simulink model "PulsePairProc"  (Simulink 6.4)
settings: Solver=ode45  StartTime=0.0  StopTime=40000/12e6  RelTol=1e-3
libraries: xbsIndex_r4 x256, simulink x2, dspsrcs4 x1
(part 2 of 2)

== system PulsePairProc/Pulse Pair Processor/Sum/A Avg/Avg. A 2 ==
  In : Inport
  M : Inport  Port=2
  N : Inport  Port=3
  Gate : Inport  Port=4
  Reset : Inport  Port=5
  AddSub2 : xbsIndex_r4/AddSub  mode=Addition  use_carryin=off  use_carryout=off  en=off  latency=0  precision=User Defined  arith_type="Signed  (2's comp)"  n_bits=33  bin_pt=31  quantization="Round  (unbiased: +/- Inf)"  overflow=Flag as error  dbl_ovrd=off  use_behavioral_HDL=off  pipelined=on  use_rpm=on  block_type=addsub
      settings: block_version=8.2
  Delay : xbsIndex_r4/Delay  en=off  latency=1  dbl_ovrd=off  reg_retiming=off  block_type=delay
      settings: infoedit=Hardware notes: A delay line is a chain, each link of which is an SRL16 followed by a flip-flop. If register retiming is enabled, the delay line is a chain of flip-flops.  block_version=8.2
  Delay1 : xbsIndex_r4/Delay  en=off  latency=1  dbl_ovrd=off  reg_retiming=off  block_type=delay
      settings: infoedit=Hardware notes: A delay line is a chain, each link of which is an SRL16 followed by a flip-flop. If register retiming is enabled, the delay line is a chain of flip-flops.  block_version=8.2
  FIFO : xbsIndex_r4/FIFO  depth=1K  percent_nbits=1  rst=on  en=off  dbl_ovrd=off  mem_type=Block RAM  block_type=fifo
      settings: block_version=8.2
  Logical : xbsIndex_r4/Logical  logical_function=OR  inputs=2  en=off  latency=0  precision=Full  arith_type=Unsigned  n_bits=16  bin_pt=0  align_bp=on  dbl_ovrd=off  block_type=logical
      settings: block_version=8.2
  Logical4 : xbsIndex_r4/Logical  logical_function=OR  inputs=2  en=off  latency=0  precision=Full  arith_type=Unsigned  n_bits=16  bin_pt=0  align_bp=on  dbl_ovrd=off  block_type=logical
      settings: block_version=8.2
  Mux : xbsIndex_r4/Mux  inputs=2  en=off  latency=0  precision=Full  arith_type=Unsigned  n_bits=16  bin_pt=14  quantization=Truncate  overflow=Wrap  dbl_ovrd=off  block_type=mux
      settings: block_version=8.2
  Register : xbsIndex_r4/Register  init=0  rst=on  en=on  dbl_ovrd=off  block_type=register
      settings: block_version=8.2
  Register1 : xbsIndex_r4/Register  init=0  rst=on  en=off  dbl_ovrd=off  block_type=register
      settings: block_version=8.2
  Shift : xbsIndex_r4/Shift  shift_dir=Right  shift_bits=1  en=off  latency=0  precision=User Defined  arith_type="Signed  (2's comp)"  n_bits=32  bin_pt=31  quantization="Round  (unbiased: +/- Inf)"  overflow=Flag as error  dbl_ovrd=off  block_type=shift
      settings: block_version=8.2
  Subsystem : Subsystem
  Out : Outport
  A,B,P Gate 1 : Outport  Port=2
  wires:
  Subsystem/1(WE) -> FIFO/2
  Subsystem/2(RE) -> Register1/1, FIFO/3
  Mux/1 -> FIFO/1, Register/1
  AddSub2/1 -> Shift/1
  FIFO/1 -> AddSub2/1
  Register1/1 -> Mux/1
  In/1 -> Delay/1
  Register/1 -> Out/1
  M/1 -> Subsystem/2(M)
  Subsystem/4(Out_En) -> Register/3, Delay1/1, Logical/2
  N/1 -> Subsystem/3(N)
  Delay/1 -> Mux/2, AddSub2/2
  Gate/1 -> Subsystem/1(Enable)
  Delay1/1 -> Logical/1
  Logical/1 -> A,B,P Gate 1/1
  Reset/1 -> Subsystem/4(Reset), Logical4/2, FIFO/4
  Logical4/1 -> Register1/2, Register/2
  Subsystem/3(RST) -> Logical4/1
  Shift/1 -> Mux/3

== system PulsePairProc/Pulse Pair Processor/Sum/B Avg/Avg. B 1 ==
  In : Inport
  M : Inport  Port=2
  N : Inport  Port=3
  Gate : Inport  Port=4
  Reset : Inport  Port=5
  AddSub2 : xbsIndex_r4/AddSub  mode=Addition  use_carryin=off  use_carryout=off  en=off  latency=0  precision=User Defined  arith_type="Signed  (2's comp)"  n_bits=33  bin_pt=31  quantization="Round  (unbiased: +/- Inf)"  overflow=Flag as error  dbl_ovrd=off  use_behavioral_HDL=off  pipelined=on  use_rpm=on  block_type=addsub
      settings: block_version=8.2
  Delay : xbsIndex_r4/Delay  en=off  latency=1  dbl_ovrd=off  reg_retiming=off  block_type=delay
      settings: infoedit=Hardware notes: A delay line is a chain, each link of which is an SRL16 followed by a flip-flop. If register retiming is enabled, the delay line is a chain of flip-flops.  block_version=8.2
  FIFO : xbsIndex_r4/FIFO  depth=1K  percent_nbits=1  rst=on  en=off  dbl_ovrd=off  mem_type=Block RAM  block_type=fifo
      settings: block_version=8.2
  Logical4 : xbsIndex_r4/Logical  logical_function=OR  inputs=2  en=off  latency=0  precision=Full  arith_type=Unsigned  n_bits=16  bin_pt=0  align_bp=on  dbl_ovrd=off  block_type=logical
      settings: block_version=8.2
  Mux : xbsIndex_r4/Mux  inputs=2  en=off  latency=0  precision=Full  arith_type=Unsigned  n_bits=16  bin_pt=14  quantization=Truncate  overflow=Wrap  dbl_ovrd=off  block_type=mux
      settings: block_version=8.2
  Register : xbsIndex_r4/Register  init=0  rst=on  en=on  dbl_ovrd=off  block_type=register
      settings: block_version=8.2
  Register1 : xbsIndex_r4/Register  init=0  rst=on  en=off  dbl_ovrd=off  block_type=register
      settings: block_version=8.2
  Shift : xbsIndex_r4/Shift  shift_dir=Right  shift_bits=1  en=off  latency=0  precision=User Defined  arith_type="Signed  (2's comp)"  n_bits=32  bin_pt=31  quantization="Round  (unbiased: +/- Inf)"  overflow=Flag as error  dbl_ovrd=off  block_type=shift
      settings: block_version=8.2
  Subsystem : Subsystem
  Out : Outport
  wires:
  Subsystem/1(WE) -> FIFO/2
  Subsystem/2(RE) -> Register1/1, FIFO/3
  Mux/1 -> FIFO/1, Register/1
  AddSub2/1 -> Shift/1
  FIFO/1 -> AddSub2/1
  Register1/1 -> Mux/1
  In/1 -> Delay/1
  Register/1 -> Out/1
  M/1 -> Subsystem/2(M)
  Subsystem/4(Out_En) -> Register/3
  N/1 -> Subsystem/3(N)
  Delay/1 -> Mux/2, AddSub2/2
  Gate/1 -> Subsystem/1(Enable)
  Reset/1 -> Subsystem/4(Reset), Logical4/2, FIFO/4
  Logical4/1 -> Register1/2, Register/2
  Subsystem/3(RST) -> Logical4/1
  Shift/1 -> Mux/3

== system PulsePairProc/Pulse Pair Processor/Sum/B Avg/Avg. B 2 ==
  In : Inport
  M : Inport  Port=2
  N : Inport  Port=3
  Gate : Inport  Port=4
  Reset : Inport  Port=5
  AddSub2 : xbsIndex_r4/AddSub  mode=Addition  use_carryin=off  use_carryout=off  en=off  latency=0  precision=User Defined  arith_type="Signed  (2's comp)"  n_bits=33  bin_pt=31  quantization="Round  (unbiased: +/- Inf)"  overflow=Flag as error  dbl_ovrd=off  use_behavioral_HDL=off  pipelined=on  use_rpm=on  block_type=addsub
      settings: block_version=8.2
  Delay : xbsIndex_r4/Delay  en=off  latency=1  dbl_ovrd=off  reg_retiming=off  block_type=delay
      settings: infoedit=Hardware notes: A delay line is a chain, each link of which is an SRL16 followed by a flip-flop. If register retiming is enabled, the delay line is a chain of flip-flops.  block_version=8.2
  FIFO : xbsIndex_r4/FIFO  depth=1K  percent_nbits=1  rst=on  en=off  dbl_ovrd=off  mem_type=Block RAM  block_type=fifo
      settings: block_version=8.2
  Logical4 : xbsIndex_r4/Logical  logical_function=OR  inputs=2  en=off  latency=0  precision=Full  arith_type=Unsigned  n_bits=16  bin_pt=0  align_bp=on  dbl_ovrd=off  block_type=logical
      settings: block_version=8.2
  Mux : xbsIndex_r4/Mux  inputs=2  en=off  latency=0  precision=Full  arith_type=Unsigned  n_bits=16  bin_pt=14  quantization=Truncate  overflow=Wrap  dbl_ovrd=off  block_type=mux
      settings: block_version=8.2
  Register : xbsIndex_r4/Register  init=0  rst=on  en=on  dbl_ovrd=off  block_type=register
      settings: block_version=8.2
  Register1 : xbsIndex_r4/Register  init=0  rst=on  en=off  dbl_ovrd=off  block_type=register
      settings: block_version=8.2
  Shift : xbsIndex_r4/Shift  shift_dir=Right  shift_bits=1  en=off  latency=0  precision=User Defined  arith_type="Signed  (2's comp)"  n_bits=32  bin_pt=31  quantization="Round  (unbiased: +/- Inf)"  overflow=Flag as error  dbl_ovrd=off  block_type=shift
      settings: block_version=8.2
  Subsystem : Subsystem
  Out : Outport
  wires:
  Subsystem/1(WE) -> FIFO/2
  Subsystem/2(RE) -> Register1/1, FIFO/3
  Mux/1 -> FIFO/1, Register/1
  AddSub2/1 -> Shift/1
  FIFO/1 -> AddSub2/1
  Register1/1 -> Mux/1
  In/1 -> Delay/1
  Register/1 -> Out/1
  M/1 -> Subsystem/2(M)
  Subsystem/4(Out_En) -> Register/3
  N/1 -> Subsystem/3(N)
  Delay/1 -> Mux/2, AddSub2/2
  Gate/1 -> Subsystem/1(Enable)
  Reset/1 -> Subsystem/4(Reset), Logical4/2, FIFO/4
  Logical4/1 -> Register1/2, Register/2
  Subsystem/3(RST) -> Logical4/1
  Shift/1 -> Mux/3

== system PulsePairProc/Pulse Pair Processor/Sum/P Avg/Avg. P 1 ==
  In : Inport
  M : Inport  Port=2
  N : Inport  Port=3
  Gate : Inport  Port=4
  Reset : Inport  Port=5
  AddSub1 : xbsIndex_r4/AddSub  mode=Addition  use_carryin=off  use_carryout=off  en=off  latency=0  precision=User Defined  arith_type=Unsigned  n_bits=33  bin_pt=32  quantization="Round  (unbiased: +/- Inf)"  overflow=Flag as error  dbl_ovrd=off  use_behavioral_HDL=off  pipelined=on  use_rpm=on  block_type=addsub
      settings: block_version=8.2
  Delay1 : xbsIndex_r4/Delay  en=off  latency=1  dbl_ovrd=off  reg_retiming=off  block_type=delay
      settings: infoedit=Hardware notes: A delay line is a chain, each link of which is an SRL16 followed by a flip-flop. If register retiming is enabled, the delay line is a chain of flip-flops.  block_version=8.2
  FIFO : xbsIndex_r4/FIFO  depth=1K  percent_nbits=1  rst=on  en=off  dbl_ovrd=off  mem_type=Block RAM  block_type=fifo
      settings: block_version=8.2
  Logical4 : xbsIndex_r4/Logical  logical_function=OR  inputs=2  en=off  latency=0  precision=Full  arith_type=Unsigned  n_bits=16  bin_pt=0  align_bp=on  dbl_ovrd=off  block_type=logical
      settings: block_version=8.2
  Mux : xbsIndex_r4/Mux  inputs=2  en=off  latency=0  precision=Full  arith_type=Unsigned  n_bits=16  bin_pt=14  quantization=Truncate  overflow=Wrap  dbl_ovrd=off  block_type=mux
      settings: block_version=8.2
  Register : xbsIndex_r4/Register  init=0  rst=on  en=on  dbl_ovrd=off  block_type=register
      settings: block_version=8.2
  Register1 : xbsIndex_r4/Register  init=0  rst=on  en=off  dbl_ovrd=off  block_type=register
      settings: block_version=8.2
  Shift : xbsIndex_r4/Shift  shift_dir=Right  shift_bits=1  en=off  latency=0  precision=User Defined  arith_type=Unsigned  n_bits=32  bin_pt=32  quantization="Round  (unbiased: +/- Inf)"  overflow=Flag as error  dbl_ovrd=off  block_type=shift
      settings: block_version=8.2
  Subsystem : Subsystem
  Out : Outport
  wires:
  Subsystem/1(WE) -> FIFO/2
  Subsystem/2(RE) -> Register1/1, FIFO/3
  Mux/1 -> FIFO/1, Register/1
  AddSub1/1 -> Shift/1
  FIFO/1 -> AddSub1/1
  Register1/1 -> Mux/1
  In/1 -> Delay1/1
  Register/1 -> Out/1
  M/1 -> Subsystem/2(M)
  Subsystem/4(Out_En) -> Register/3
  N/1 -> Subsystem/3(N)
  Delay1/1 -> AddSub1/2, Mux/2
  Gate/1 -> Subsystem/1(Enable)
  Reset/1 -> Subsystem/4(Reset), Logical4/2, FIFO/4
  Logical4/1 -> Register1/2, Register/2
  Subsystem/3(RST) -> Logical4/1
  Shift/1 -> Mux/3

== system PulsePairProc/Pulse Pair Processor/Sum/P Avg/Avg. P 2 ==
  In : Inport
  M : Inport  Port=2
  N : Inport  Port=3
  Gate : Inport  Port=4
  Reset : Inport  Port=5
  AddSub1 : xbsIndex_r4/AddSub  mode=Addition  use_carryin=off  use_carryout=off  en=off  latency=0  precision=User Defined  arith_type=Unsigned  n_bits=33  bin_pt=32  quantization="Round  (unbiased: +/- Inf)"  overflow=Flag as error  dbl_ovrd=off  use_behavioral_HDL=off  pipelined=on  use_rpm=on  block_type=addsub
      settings: block_version=8.2
  Delay1 : xbsIndex_r4/Delay  en=off  latency=1  dbl_ovrd=off  reg_retiming=off  block_type=delay
      settings: infoedit=Hardware notes: A delay line is a chain, each link of which is an SRL16 followed by a flip-flop. If register retiming is enabled, the delay line is a chain of flip-flops.  block_version=8.2
  FIFO : xbsIndex_r4/FIFO  depth=1K  percent_nbits=1  rst=on  en=off  dbl_ovrd=off  mem_type=Block RAM  block_type=fifo
      settings: block_version=8.2
  Logical4 : xbsIndex_r4/Logical  logical_function=OR  inputs=2  en=off  latency=0  precision=Full  arith_type=Unsigned  n_bits=16  bin_pt=0  align_bp=on  dbl_ovrd=off  block_type=logical
      settings: block_version=8.2
  Mux : xbsIndex_r4/Mux  inputs=2  en=off  latency=0  precision=Full  arith_type=Unsigned  n_bits=16  bin_pt=14  quantization=Truncate  overflow=Wrap  dbl_ovrd=off  block_type=mux
      settings: block_version=8.2
  Register : xbsIndex_r4/Register  init=0  rst=on  en=on  dbl_ovrd=off  block_type=register
      settings: block_version=8.2
  Register1 : xbsIndex_r4/Register  init=0  rst=on  en=off  dbl_ovrd=off  block_type=register
      settings: block_version=8.2
  Shift1 : xbsIndex_r4/Shift  shift_dir=Right  shift_bits=1  en=off  latency=0  precision=User Defined  arith_type=Unsigned  n_bits=32  bin_pt=32  quantization="Round  (unbiased: +/- Inf)"  overflow=Flag as error  dbl_ovrd=off  block_type=shift
      settings: block_version=8.2
  Subsystem : Subsystem
  Out : Outport
  wires:
  Subsystem/1(WE) -> FIFO/2
  Subsystem/2(RE) -> Register1/1, FIFO/3
  Mux/1 -> FIFO/1, Register/1
  AddSub1/1 -> Shift1/1
  FIFO/1 -> AddSub1/1
  Register1/1 -> Mux/1
  In/1 -> Delay1/1
  Register/1 -> Out/1
  M/1 -> Subsystem/2(M)
  Subsystem/4(Out_En) -> Register/3
  N/1 -> Subsystem/3(N)
  Delay1/1 -> AddSub1/2, Mux/2
  Gate/1 -> Subsystem/1(Enable)
  Reset/1 -> Subsystem/4(Reset), Logical4/2, FIFO/4
  Logical4/1 -> Register1/2, Register/2
  Subsystem/3(RST) -> Logical4/1
  Shift1/1 -> Mux/3

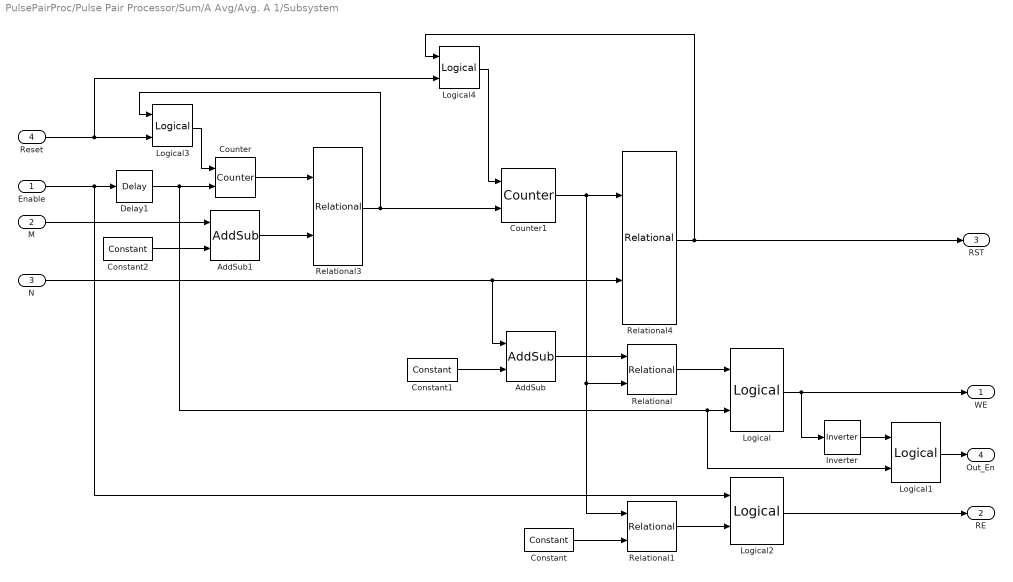
== system PulsePairProc/Pulse Pair Processor/Sum/A Avg/Avg. A 1/Subsystem ==
  Enable : Inport
  M : Inport  Port=2
  N : Inport  Port=3
  Reset : Inport  Port=4
  AddSub : xbsIndex_r4/AddSub  mode=Subtraction  use_carryin=off  use_carryout=off  en=off  latency=0  precision=User Defined  arith_type=Unsigned  n_bits=7  bin_pt=0  quantization="Round  (unbiased: +/- Inf)"  overflow=Flag as error  dbl_ovrd=off  use_behavioral_HDL=off  pipelined=off  use_rpm=on  block_type=addsub
      settings: block_version=8.2
  AddSub1 : xbsIndex_r4/AddSub  mode=Subtraction  use_carryin=off  use_carryout=off  en=off  latency=0  precision=User Defined  arith_type=Unsigned  n_bits=11  bin_pt=0  quantization="Round  (unbiased: +/- Inf)"  overflow=Flag as error  dbl_ovrd=off  use_behavioral_HDL=off  pipelined=off  use_rpm=on  block_type=addsub
      settings: block_version=8.2
  Constant : xbsIndex_r4/Constant  arith_type=Unsigned  const=0  n_bits=1  bin_pt=0  explicit_period=off  period=1  equ=P=C  opselect=C  inp2=PCIN>>17  opr=+  inp1=P  carry=CIN  dbl_ovrd=off  block_type=constant
      settings: block_version=8.2
  Constant1 : xbsIndex_r4/Constant  arith_type=Unsigned  const=1  n_bits=1  bin_pt=0  explicit_period=off  period=1  equ=P=C  opselect=C  inp2=PCIN>>17  opr=+  inp1=P  carry=CIN  dbl_ovrd=off  block_type=constant
      settings: block_version=8.2
  Constant2 : xbsIndex_r4/Constant  arith_type=Unsigned  const=1  n_bits=1  bin_pt=0  explicit_period=off  period=1  equ=P=C  opselect=C  inp2=PCIN>>17  opr=+  inp1=P  carry=CIN  dbl_ovrd=off  block_type=constant
      settings: block_version=8.2
  Counter : xbsIndex_r4/Counter  cnt_type=Count Limited  cnt_to=2047  operation=Up  start_count=0  cnt_by_val=1  arith_type=Unsigned  n_bits=11  bin_pt=0  load_pin=off  rst=on  en=on  explicit_period=on  period=1/12e6  dbl_ovrd=off  use_behavioral_HDL=off  use_rpm=off  block_type=counter
      settings: block_version=8.2
  Counter1 : xbsIndex_r4/Counter  cnt_type=Count Limited  cnt_to=127  operation=Up  start_count=0  cnt_by_val=1  arith_type=Unsigned  n_bits=7  bin_pt=0  load_pin=off  rst=on  en=on  explicit_period=on  period=1/12e6  dbl_ovrd=off  use_behavioral_HDL=off  use_rpm=off  block_type=counter
      settings: block_version=8.2
  Delay1 : xbsIndex_r4/Delay  en=off  latency=1  dbl_ovrd=off  reg_retiming=off  block_type=delay
      settings: infoedit=Hardware notes: A delay line is a chain, each link of which is an SRL16 followed by a flip-flop. If register retiming is enabled, the delay line is a chain of flip-flops.  block_version=8.2
  Inverter : xbsIndex_r4/Inverter  en=off  latency=0  dbl_ovrd=off  block_type=inv
      settings: block_version=8.2
  Logical : xbsIndex_r4/Logical  logical_function=AND  inputs=2  en=off  latency=0  precision=Full  arith_type=Unsigned  n_bits=16  bin_pt=0  align_bp=on  dbl_ovrd=off  block_type=logical
      settings: block_version=8.2
  Logical1 : xbsIndex_r4/Logical  logical_function=AND  inputs=2  en=off  latency=0  precision=Full  arith_type=Unsigned  n_bits=16  bin_pt=0  align_bp=on  dbl_ovrd=off  block_type=logical
      settings: block_version=8.2
  Logical2 : xbsIndex_r4/Logical  logical_function=AND  inputs=2  en=off  latency=0  precision=Full  arith_type=Unsigned  n_bits=16  bin_pt=0  align_bp=on  dbl_ovrd=off  block_type=logical
      settings: block_version=8.2
  Logical3 : xbsIndex_r4/Logical  logical_function=OR  inputs=2  en=off  latency=0  precision=Full  arith_type=Unsigned  n_bits=16  bin_pt=0  align_bp=on  dbl_ovrd=off  block_type=logical
      settings: block_version=8.2
  Logical4 : xbsIndex_r4/Logical  logical_function=OR  inputs=2  en=off  latency=0  precision=Full  arith_type=Unsigned  n_bits=16  bin_pt=0  align_bp=on  dbl_ovrd=off  block_type=logical
      settings: block_version=8.2
  Relational : xbsIndex_r4/Relational  mode=a!=b  en=off  latency=0  dbl_ovrd=off  block_type=relational
      settings: block_version=8.2
  Relational1 : xbsIndex_r4/Relational  mode=a!=b  en=off  latency=0  dbl_ovrd=off  block_type=relational
      settings: block_version=8.2
  Relational3 : xbsIndex_r4/Relational  mode=a=b  en=off  latency=0  dbl_ovrd=off  block_type=relational
      settings: block_version=8.2
  Relational4 : xbsIndex_r4/Relational  mode=a=b  en=off  latency=0  dbl_ovrd=off  block_type=relational
      settings: block_version=8.2
  WE : Outport
  RE : Outport  Port=2
  RST : Outport  Port=3
  Out_En : Outport  Port=4
  wires:
  Logical1/1 -> Out_En/1
  Logical2/1 -> RE/1
  Enable/1 -> Delay1/1, Logical2/1
  Counter/1 -> Relational3/1
  Relational3/1 -> Counter1/2, Logical3/1
  Counter1/1 -> Relational4/1, Relational/2, Relational1/1
  N/1 -> Relational4/2, AddSub/1
  Relational4/1 -> RST/1, Logical4/1
  Relational/1 -> Logical/1
  Logical/1 -> WE/1, Inverter/1
  Inverter/1 -> Logical1/1
  Constant/1 -> Relational1/2
  Relational1/1 -> Logical2/2
  Delay1/1 -> Counter/2, Logical/2, Logical1/2
  Constant1/1 -> AddSub/2
  Constant2/1 -> AddSub1/2
  AddSub1/1 -> Relational3/2
  M/1 -> AddSub1/1
  AddSub/1 -> Relational/1
  Logical3/1 -> Counter/1
  Reset/1 -> Logical3/2, Logical4/2
  Logical4/1 -> Counter1/1

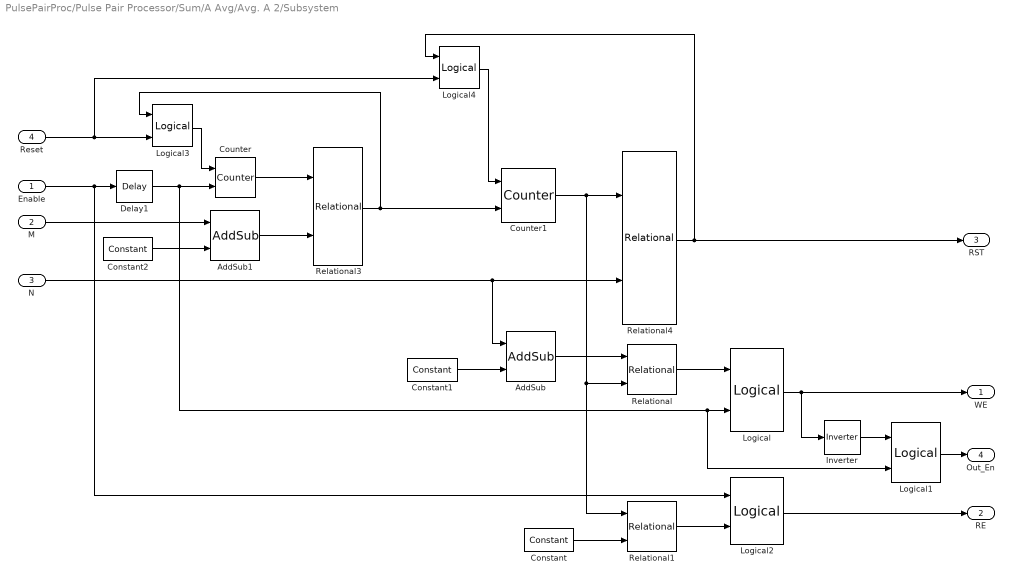
== system PulsePairProc/Pulse Pair Processor/Sum/A Avg/Avg. A 2/Subsystem ==
  Enable : Inport
  M : Inport  Port=2
  N : Inport  Port=3
  Reset : Inport  Port=4
  AddSub : xbsIndex_r4/AddSub  mode=Subtraction  use_carryin=off  use_carryout=off  en=off  latency=0  precision=User Defined  arith_type=Unsigned  n_bits=7  bin_pt=0  quantization="Round  (unbiased: +/- Inf)"  overflow=Flag as error  dbl_ovrd=off  use_behavioral_HDL=off  pipelined=off  use_rpm=on  block_type=addsub
      settings: block_version=8.2
  AddSub1 : xbsIndex_r4/AddSub  mode=Subtraction  use_carryin=off  use_carryout=off  en=off  latency=0  precision=User Defined  arith_type=Unsigned  n_bits=11  bin_pt=0  quantization="Round  (unbiased: +/- Inf)"  overflow=Flag as error  dbl_ovrd=off  use_behavioral_HDL=off  pipelined=off  use_rpm=on  block_type=addsub
      settings: block_version=8.2
  Constant : xbsIndex_r4/Constant  arith_type=Unsigned  const=0  n_bits=1  bin_pt=0  explicit_period=off  period=1  equ=P=C  opselect=C  inp2=PCIN>>17  opr=+  inp1=P  carry=CIN  dbl_ovrd=off  block_type=constant
      settings: block_version=8.2
  Constant1 : xbsIndex_r4/Constant  arith_type=Unsigned  const=1  n_bits=1  bin_pt=0  explicit_period=off  period=1  equ=P=C  opselect=C  inp2=PCIN>>17  opr=+  inp1=P  carry=CIN  dbl_ovrd=off  block_type=constant
      settings: block_version=8.2
  Constant2 : xbsIndex_r4/Constant  arith_type=Unsigned  const=1  n_bits=1  bin_pt=0  explicit_period=off  period=1  equ=P=C  opselect=C  inp2=PCIN>>17  opr=+  inp1=P  carry=CIN  dbl_ovrd=off  block_type=constant
      settings: block_version=8.2
  Counter : xbsIndex_r4/Counter  cnt_type=Free Running  cnt_to=11  operation=Up  start_count=0  cnt_by_val=1  arith_type=Unsigned  n_bits=11  bin_pt=0  load_pin=off  rst=on  en=on  explicit_period=on  period=1/12e6  dbl_ovrd=off  use_behavioral_HDL=off  use_rpm=off  block_type=counter
      settings: block_version=8.2
  Counter1 : xbsIndex_r4/Counter  cnt_type=Free Running  cnt_to=Inf  operation=Up  start_count=0  cnt_by_val=1  arith_type=Unsigned  n_bits=7  bin_pt=0  load_pin=off  rst=on  en=on  explicit_period=on  period=1/12e6  dbl_ovrd=off  use_behavioral_HDL=off  use_rpm=off  block_type=counter
      settings: block_version=8.2
  Delay1 : xbsIndex_r4/Delay  en=off  latency=1  dbl_ovrd=off  reg_retiming=off  block_type=delay
      settings: infoedit=Hardware notes: A delay line is a chain, each link of which is an SRL16 followed by a flip-flop. If register retiming is enabled, the delay line is a chain of flip-flops.  block_version=8.2
  Inverter : xbsIndex_r4/Inverter  en=off  latency=0  dbl_ovrd=off  block_type=inv
      settings: block_version=8.2
  Logical : xbsIndex_r4/Logical  logical_function=AND  inputs=2  en=off  latency=0  precision=Full  arith_type=Unsigned  n_bits=16  bin_pt=0  align_bp=on  dbl_ovrd=off  block_type=logical
      settings: block_version=8.2
  Logical1 : xbsIndex_r4/Logical  logical_function=AND  inputs=2  en=off  latency=0  precision=Full  arith_type=Unsigned  n_bits=16  bin_pt=0  align_bp=on  dbl_ovrd=off  block_type=logical
      settings: block_version=8.2
  Logical2 : xbsIndex_r4/Logical  logical_function=AND  inputs=2  en=off  latency=0  precision=Full  arith_type=Unsigned  n_bits=16  bin_pt=0  align_bp=on  dbl_ovrd=off  block_type=logical
      settings: block_version=8.2
  Logical3 : xbsIndex_r4/Logical  logical_function=OR  inputs=2  en=off  latency=0  precision=Full  arith_type=Unsigned  n_bits=16  bin_pt=0  align_bp=on  dbl_ovrd=off  block_type=logical
      settings: block_version=8.2
  Logical4 : xbsIndex_r4/Logical  logical_function=OR  inputs=2  en=off  latency=0  precision=Full  arith_type=Unsigned  n_bits=16  bin_pt=0  align_bp=on  dbl_ovrd=off  block_type=logical
      settings: block_version=8.2
  Relational : xbsIndex_r4/Relational  mode=a!=b  en=off  latency=0  dbl_ovrd=off  block_type=relational
      settings: block_version=8.2
  Relational1 : xbsIndex_r4/Relational  mode=a!=b  en=off  latency=0  dbl_ovrd=off  block_type=relational
      settings: block_version=8.2
  Relational3 : xbsIndex_r4/Relational  mode=a=b  en=off  latency=0  dbl_ovrd=off  block_type=relational
      settings: block_version=8.2
  Relational4 : xbsIndex_r4/Relational  mode=a=b  en=off  latency=0  dbl_ovrd=off  block_type=relational
      settings: block_version=8.2
  WE : Outport
  RE : Outport  Port=2
  RST : Outport  Port=3
  Out_En : Outport  Port=4
  wires:
  Logical1/1 -> Out_En/1
  Logical2/1 -> RE/1
  Enable/1 -> Delay1/1, Logical2/1
  Counter/1 -> Relational3/1
  Relational3/1 -> Counter1/2, Logical3/1
  Counter1/1 -> Relational4/1, Relational/2, Relational1/1
  N/1 -> Relational4/2, AddSub/1
  Relational4/1 -> RST/1, Logical4/1
  Relational/1 -> Logical/1
  Logical/1 -> WE/1, Inverter/1
  Inverter/1 -> Logical1/1
  Constant/1 -> Relational1/2
  Relational1/1 -> Logical2/2
  Delay1/1 -> Counter/2, Logical/2, Logical1/2
  Constant1/1 -> AddSub/2
  Constant2/1 -> AddSub1/2
  AddSub1/1 -> Relational3/2
  M/1 -> AddSub1/1
  AddSub/1 -> Relational/1
  Logical3/1 -> Counter/1
  Reset/1 -> Logical3/2, Logical4/2
  Logical4/1 -> Counter1/1

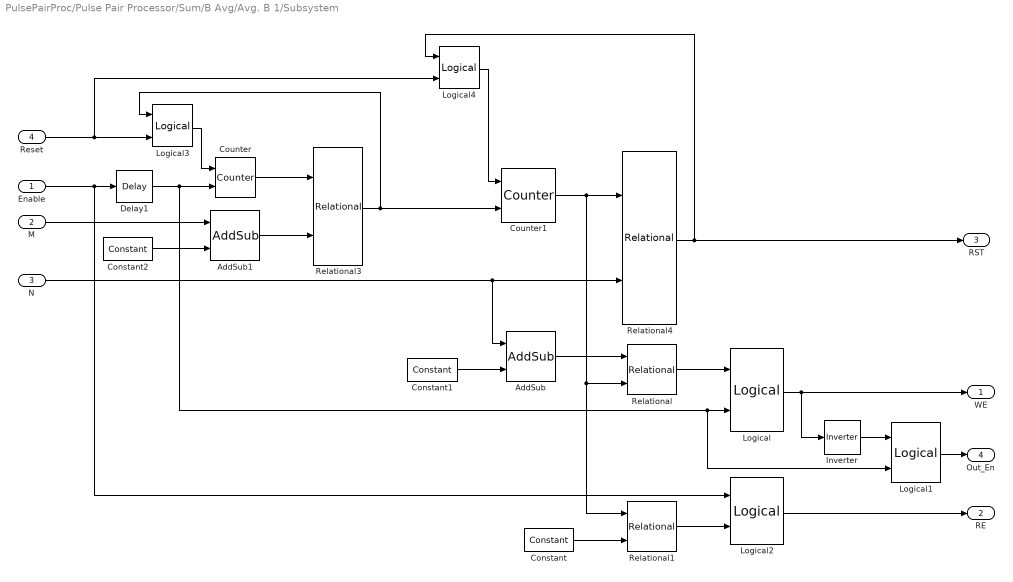
== system PulsePairProc/Pulse Pair Processor/Sum/B Avg/Avg. B 1/Subsystem ==
  Enable : Inport
  M : Inport  Port=2
  N : Inport  Port=3
  Reset : Inport  Port=4
  AddSub : xbsIndex_r4/AddSub  mode=Subtraction  use_carryin=off  use_carryout=off  en=off  latency=0  precision=User Defined  arith_type=Unsigned  n_bits=7  bin_pt=0  quantization="Round  (unbiased: +/- Inf)"  overflow=Flag as error  dbl_ovrd=off  use_behavioral_HDL=off  pipelined=off  use_rpm=on  block_type=addsub
      settings: block_version=8.2
  AddSub1 : xbsIndex_r4/AddSub  mode=Subtraction  use_carryin=off  use_carryout=off  en=off  latency=0  precision=User Defined  arith_type=Unsigned  n_bits=11  bin_pt=0  quantization="Round  (unbiased: +/- Inf)"  overflow=Flag as error  dbl_ovrd=off  use_behavioral_HDL=off  pipelined=off  use_rpm=on  block_type=addsub
      settings: block_version=8.2
  Constant : xbsIndex_r4/Constant  arith_type=Unsigned  const=0  n_bits=1  bin_pt=0  explicit_period=off  period=1  equ=P=C  opselect=C  inp2=PCIN>>17  opr=+  inp1=P  carry=CIN  dbl_ovrd=off  block_type=constant
      settings: block_version=8.2
  Constant1 : xbsIndex_r4/Constant  arith_type=Unsigned  const=1  n_bits=1  bin_pt=0  explicit_period=off  period=1  equ=P=C  opselect=C  inp2=PCIN>>17  opr=+  inp1=P  carry=CIN  dbl_ovrd=off  block_type=constant
      settings: block_version=8.2
  Constant2 : xbsIndex_r4/Constant  arith_type=Unsigned  const=1  n_bits=1  bin_pt=0  explicit_period=off  period=1  equ=P=C  opselect=C  inp2=PCIN>>17  opr=+  inp1=P  carry=CIN  dbl_ovrd=off  block_type=constant
      settings: block_version=8.2
  Counter : xbsIndex_r4/Counter  cnt_type=Free Running  cnt_to=11  operation=Up  start_count=0  cnt_by_val=1  arith_type=Unsigned  n_bits=11  bin_pt=0  load_pin=off  rst=on  en=on  explicit_period=on  period=1/12e6  dbl_ovrd=off  use_behavioral_HDL=off  use_rpm=off  block_type=counter
      settings: block_version=8.2
  Counter1 : xbsIndex_r4/Counter  cnt_type=Free Running  cnt_to=Inf  operation=Up  start_count=0  cnt_by_val=1  arith_type=Unsigned  n_bits=7  bin_pt=0  load_pin=off  rst=on  en=on  explicit_period=on  period=1/12e6  dbl_ovrd=off  use_behavioral_HDL=off  use_rpm=off  block_type=counter
      settings: block_version=8.2
  Delay1 : xbsIndex_r4/Delay  en=off  latency=1  dbl_ovrd=off  reg_retiming=off  block_type=delay
      settings: infoedit=Hardware notes: A delay line is a chain, each link of which is an SRL16 followed by a flip-flop. If register retiming is enabled, the delay line is a chain of flip-flops.  block_version=8.2
  Inverter : xbsIndex_r4/Inverter  en=off  latency=0  dbl_ovrd=off  block_type=inv
      settings: block_version=8.2
  Logical : xbsIndex_r4/Logical  logical_function=AND  inputs=2  en=off  latency=0  precision=Full  arith_type=Unsigned  n_bits=16  bin_pt=0  align_bp=on  dbl_ovrd=off  block_type=logical
      settings: block_version=8.2
  Logical1 : xbsIndex_r4/Logical  logical_function=AND  inputs=2  en=off  latency=0  precision=Full  arith_type=Unsigned  n_bits=16  bin_pt=0  align_bp=on  dbl_ovrd=off  block_type=logical
      settings: block_version=8.2
  Logical2 : xbsIndex_r4/Logical  logical_function=AND  inputs=2  en=off  latency=0  precision=Full  arith_type=Unsigned  n_bits=16  bin_pt=0  align_bp=on  dbl_ovrd=off  block_type=logical
      settings: block_version=8.2
  Logical3 : xbsIndex_r4/Logical  logical_function=OR  inputs=2  en=off  latency=0  precision=Full  arith_type=Unsigned  n_bits=16  bin_pt=0  align_bp=on  dbl_ovrd=off  block_type=logical
      settings: block_version=8.2
  Logical4 : xbsIndex_r4/Logical  logical_function=OR  inputs=2  en=off  latency=0  precision=Full  arith_type=Unsigned  n_bits=16  bin_pt=0  align_bp=on  dbl_ovrd=off  block_type=logical
      settings: block_version=8.2
  Relational : xbsIndex_r4/Relational  mode=a!=b  en=off  latency=0  dbl_ovrd=off  block_type=relational
      settings: block_version=8.2
  Relational1 : xbsIndex_r4/Relational  mode=a!=b  en=off  latency=0  dbl_ovrd=off  block_type=relational
      settings: block_version=8.2
  Relational3 : xbsIndex_r4/Relational  mode=a=b  en=off  latency=0  dbl_ovrd=off  block_type=relational
      settings: block_version=8.2
  Relational4 : xbsIndex_r4/Relational  mode=a=b  en=off  latency=0  dbl_ovrd=off  block_type=relational
      settings: block_version=8.2
  WE : Outport
  RE : Outport  Port=2
  RST : Outport  Port=3
  Out_En : Outport  Port=4
  wires:
  Logical1/1 -> Out_En/1
  Logical2/1 -> RE/1
  Enable/1 -> Delay1/1, Logical2/1
  Counter/1 -> Relational3/1
  Relational3/1 -> Counter1/2, Logical3/1
  Counter1/1 -> Relational4/1, Relational/2, Relational1/1
  N/1 -> Relational4/2, AddSub/1
  Relational4/1 -> RST/1, Logical4/1
  Relational/1 -> Logical/1
  Logical/1 -> WE/1, Inverter/1
  Inverter/1 -> Logical1/1
  Constant/1 -> Relational1/2
  Relational1/1 -> Logical2/2
  Delay1/1 -> Counter/2, Logical/2, Logical1/2
  Constant1/1 -> AddSub/2
  Constant2/1 -> AddSub1/2
  AddSub1/1 -> Relational3/2
  M/1 -> AddSub1/1
  AddSub/1 -> Relational/1
  Logical3/1 -> Counter/1
  Reset/1 -> Logical3/2, Logical4/2
  Logical4/1 -> Counter1/1

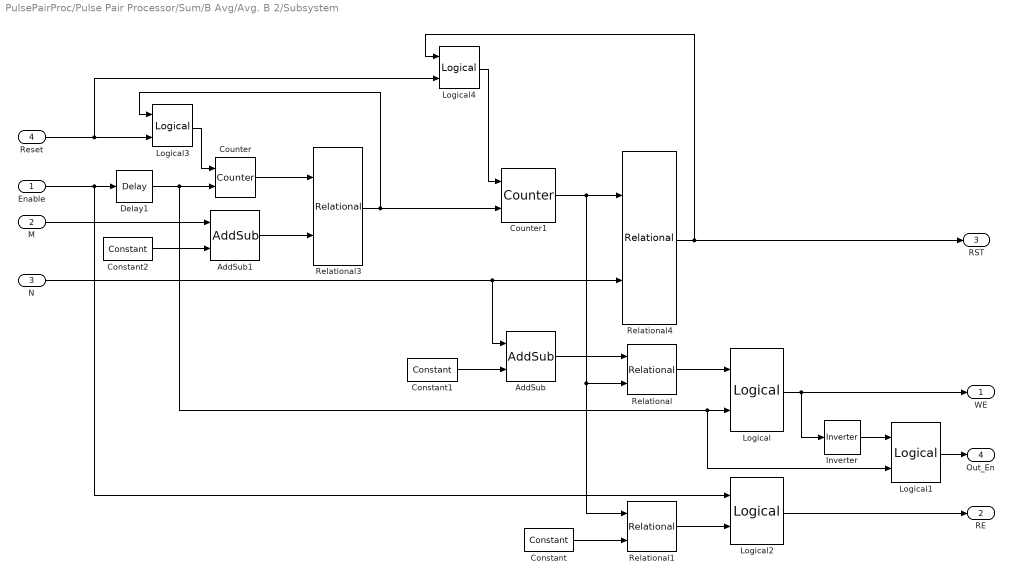
== system PulsePairProc/Pulse Pair Processor/Sum/B Avg/Avg. B 2/Subsystem ==
  Enable : Inport
  M : Inport  Port=2
  N : Inport  Port=3
  Reset : Inport  Port=4
  AddSub : xbsIndex_r4/AddSub  mode=Subtraction  use_carryin=off  use_carryout=off  en=off  latency=0  precision=User Defined  arith_type=Unsigned  n_bits=7  bin_pt=0  quantization="Round  (unbiased: +/- Inf)"  overflow=Flag as error  dbl_ovrd=off  use_behavioral_HDL=off  pipelined=off  use_rpm=on  block_type=addsub
      settings: block_version=8.2
  AddSub1 : xbsIndex_r4/AddSub  mode=Subtraction  use_carryin=off  use_carryout=off  en=off  latency=0  precision=User Defined  arith_type=Unsigned  n_bits=11  bin_pt=0  quantization="Round  (unbiased: +/- Inf)"  overflow=Flag as error  dbl_ovrd=off  use_behavioral_HDL=off  pipelined=off  use_rpm=on  block_type=addsub
      settings: block_version=8.2
  Constant : xbsIndex_r4/Constant  arith_type=Unsigned  const=0  n_bits=1  bin_pt=0  explicit_period=off  period=1  equ=P=C  opselect=C  inp2=PCIN>>17  opr=+  inp1=P  carry=CIN  dbl_ovrd=off  block_type=constant
      settings: block_version=8.2
  Constant1 : xbsIndex_r4/Constant  arith_type=Unsigned  const=1  n_bits=1  bin_pt=0  explicit_period=off  period=1  equ=P=C  opselect=C  inp2=PCIN>>17  opr=+  inp1=P  carry=CIN  dbl_ovrd=off  block_type=constant
      settings: block_version=8.2
  Constant2 : xbsIndex_r4/Constant  arith_type=Unsigned  const=1  n_bits=1  bin_pt=0  explicit_period=off  period=1  equ=P=C  opselect=C  inp2=PCIN>>17  opr=+  inp1=P  carry=CIN  dbl_ovrd=off  block_type=constant
      settings: block_version=8.2
  Counter : xbsIndex_r4/Counter  cnt_type=Free Running  cnt_to=11  operation=Up  start_count=0  cnt_by_val=1  arith_type=Unsigned  n_bits=11  bin_pt=0  load_pin=off  rst=on  en=on  explicit_period=on  period=1/12e6  dbl_ovrd=off  use_behavioral_HDL=off  use_rpm=off  block_type=counter
      settings: block_version=8.2
  Counter1 : xbsIndex_r4/Counter  cnt_type=Free Running  cnt_to=Inf  operation=Up  start_count=0  cnt_by_val=1  arith_type=Unsigned  n_bits=7  bin_pt=0  load_pin=off  rst=on  en=on  explicit_period=on  period=1/12e6  dbl_ovrd=off  use_behavioral_HDL=off  use_rpm=off  block_type=counter
      settings: block_version=8.2
  Delay1 : xbsIndex_r4/Delay  en=off  latency=1  dbl_ovrd=off  reg_retiming=off  block_type=delay
      settings: infoedit=Hardware notes: A delay line is a chain, each link of which is an SRL16 followed by a flip-flop. If register retiming is enabled, the delay line is a chain of flip-flops.  block_version=8.2
  Inverter : xbsIndex_r4/Inverter  en=off  latency=0  dbl_ovrd=off  block_type=inv
      settings: block_version=8.2
  Logical : xbsIndex_r4/Logical  logical_function=AND  inputs=2  en=off  latency=0  precision=Full  arith_type=Unsigned  n_bits=16  bin_pt=0  align_bp=on  dbl_ovrd=off  block_type=logical
      settings: block_version=8.2
  Logical1 : xbsIndex_r4/Logical  logical_function=AND  inputs=2  en=off  latency=0  precision=Full  arith_type=Unsigned  n_bits=16  bin_pt=0  align_bp=on  dbl_ovrd=off  block_type=logical
      settings: block_version=8.2
  Logical2 : xbsIndex_r4/Logical  logical_function=AND  inputs=2  en=off  latency=0  precision=Full  arith_type=Unsigned  n_bits=16  bin_pt=0  align_bp=on  dbl_ovrd=off  block_type=logical
      settings: block_version=8.2
  Logical3 : xbsIndex_r4/Logical  logical_function=OR  inputs=2  en=off  latency=0  precision=Full  arith_type=Unsigned  n_bits=16  bin_pt=0  align_bp=on  dbl_ovrd=off  block_type=logical
      settings: block_version=8.2
  Logical4 : xbsIndex_r4/Logical  logical_function=OR  inputs=2  en=off  latency=0  precision=Full  arith_type=Unsigned  n_bits=16  bin_pt=0  align_bp=on  dbl_ovrd=off  block_type=logical
      settings: block_version=8.2
  Relational : xbsIndex_r4/Relational  mode=a!=b  en=off  latency=0  dbl_ovrd=off  block_type=relational
      settings: block_version=8.2
  Relational1 : xbsIndex_r4/Relational  mode=a!=b  en=off  latency=0  dbl_ovrd=off  block_type=relational
      settings: block_version=8.2
  Relational3 : xbsIndex_r4/Relational  mode=a=b  en=off  latency=0  dbl_ovrd=off  block_type=relational
      settings: block_version=8.2
  Relational4 : xbsIndex_r4/Relational  mode=a=b  en=off  latency=0  dbl_ovrd=off  block_type=relational
      settings: block_version=8.2
  WE : Outport
  RE : Outport  Port=2
  RST : Outport  Port=3
  Out_En : Outport  Port=4
  wires:
  Logical1/1 -> Out_En/1
  Logical2/1 -> RE/1
  Enable/1 -> Delay1/1, Logical2/1
  Counter/1 -> Relational3/1
  Relational3/1 -> Counter1/2, Logical3/1
  Counter1/1 -> Relational4/1, Relational/2, Relational1/1
  N/1 -> Relational4/2, AddSub/1
  Relational4/1 -> RST/1, Logical4/1
  Relational/1 -> Logical/1
  Logical/1 -> WE/1, Inverter/1
  Inverter/1 -> Logical1/1
  Constant/1 -> Relational1/2
  Relational1/1 -> Logical2/2
  Delay1/1 -> Counter/2, Logical/2, Logical1/2
  Constant1/1 -> AddSub/2
  Constant2/1 -> AddSub1/2
  AddSub1/1 -> Relational3/2
  M/1 -> AddSub1/1
  AddSub/1 -> Relational/1
  Logical3/1 -> Counter/1
  Reset/1 -> Logical3/2, Logical4/2
  Logical4/1 -> Counter1/1

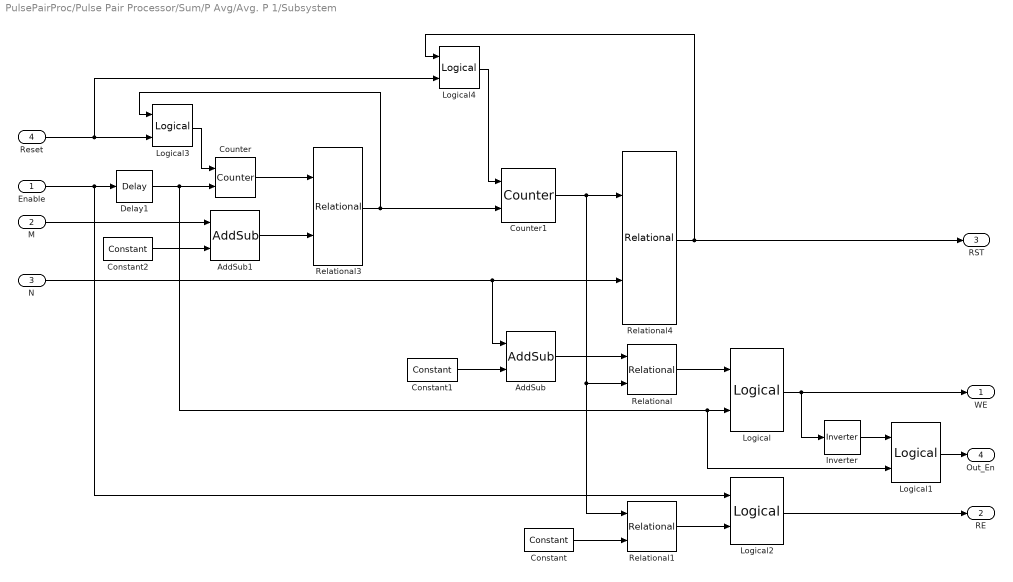
== system PulsePairProc/Pulse Pair Processor/Sum/P Avg/Avg. P 1/Subsystem ==
  Enable : Inport
  M : Inport  Port=2
  N : Inport  Port=3
  Reset : Inport  Port=4
  AddSub : xbsIndex_r4/AddSub  mode=Subtraction  use_carryin=off  use_carryout=off  en=off  latency=0  precision=User Defined  arith_type=Unsigned  n_bits=7  bin_pt=0  quantization="Round  (unbiased: +/- Inf)"  overflow=Flag as error  dbl_ovrd=off  use_behavioral_HDL=off  pipelined=off  use_rpm=on  block_type=addsub
      settings: block_version=8.2
  AddSub1 : xbsIndex_r4/AddSub  mode=Subtraction  use_carryin=off  use_carryout=off  en=off  latency=0  precision=User Defined  arith_type=Unsigned  n_bits=11  bin_pt=0  quantization="Round  (unbiased: +/- Inf)"  overflow=Flag as error  dbl_ovrd=off  use_behavioral_HDL=off  pipelined=off  use_rpm=on  block_type=addsub
      settings: block_version=8.2
  Constant : xbsIndex_r4/Constant  arith_type=Unsigned  const=0  n_bits=1  bin_pt=0  explicit_period=off  period=1  equ=P=C  opselect=C  inp2=PCIN>>17  opr=+  inp1=P  carry=CIN  dbl_ovrd=off  block_type=constant
      settings: block_version=8.2
  Constant1 : xbsIndex_r4/Constant  arith_type=Unsigned  const=1  n_bits=1  bin_pt=0  explicit_period=off  period=1  equ=P=C  opselect=C  inp2=PCIN>>17  opr=+  inp1=P  carry=CIN  dbl_ovrd=off  block_type=constant
      settings: block_version=8.2
  Constant2 : xbsIndex_r4/Constant  arith_type=Unsigned  const=1  n_bits=1  bin_pt=0  explicit_period=off  period=1  equ=P=C  opselect=C  inp2=PCIN>>17  opr=+  inp1=P  carry=CIN  dbl_ovrd=off  block_type=constant
      settings: block_version=8.2
  Counter : xbsIndex_r4/Counter  cnt_type=Free Running  cnt_to=11  operation=Up  start_count=0  cnt_by_val=1  arith_type=Unsigned  n_bits=11  bin_pt=0  load_pin=off  rst=on  en=on  explicit_period=on  period=1/12e6  dbl_ovrd=off  use_behavioral_HDL=off  use_rpm=off  block_type=counter
      settings: block_version=8.2
  Counter1 : xbsIndex_r4/Counter  cnt_type=Free Running  cnt_to=Inf  operation=Up  start_count=0  cnt_by_val=1  arith_type=Unsigned  n_bits=7  bin_pt=0  load_pin=off  rst=on  en=on  explicit_period=on  period=1/12e6  dbl_ovrd=off  use_behavioral_HDL=off  use_rpm=off  block_type=counter
      settings: block_version=8.2
  Delay1 : xbsIndex_r4/Delay  en=off  latency=1  dbl_ovrd=off  reg_retiming=off  block_type=delay
      settings: infoedit=Hardware notes: A delay line is a chain, each link of which is an SRL16 followed by a flip-flop. If register retiming is enabled, the delay line is a chain of flip-flops.  block_version=8.2
  Inverter : xbsIndex_r4/Inverter  en=off  latency=0  dbl_ovrd=off  block_type=inv
      settings: block_version=8.2
  Logical : xbsIndex_r4/Logical  logical_function=AND  inputs=2  en=off  latency=0  precision=Full  arith_type=Unsigned  n_bits=16  bin_pt=0  align_bp=on  dbl_ovrd=off  block_type=logical
      settings: block_version=8.2
  Logical1 : xbsIndex_r4/Logical  logical_function=AND  inputs=2  en=off  latency=0  precision=Full  arith_type=Unsigned  n_bits=16  bin_pt=0  align_bp=on  dbl_ovrd=off  block_type=logical
      settings: block_version=8.2
  Logical2 : xbsIndex_r4/Logical  logical_function=AND  inputs=2  en=off  latency=0  precision=Full  arith_type=Unsigned  n_bits=16  bin_pt=0  align_bp=on  dbl_ovrd=off  block_type=logical
      settings: block_version=8.2
  Logical3 : xbsIndex_r4/Logical  logical_function=OR  inputs=2  en=off  latency=0  precision=Full  arith_type=Unsigned  n_bits=16  bin_pt=0  align_bp=on  dbl_ovrd=off  block_type=logical
      settings: block_version=8.2
  Logical4 : xbsIndex_r4/Logical  logical_function=OR  inputs=2  en=off  latency=0  precision=Full  arith_type=Unsigned  n_bits=16  bin_pt=0  align_bp=on  dbl_ovrd=off  block_type=logical
      settings: block_version=8.2
  Relational : xbsIndex_r4/Relational  mode=a!=b  en=off  latency=0  dbl_ovrd=off  block_type=relational
      settings: block_version=8.2
  Relational1 : xbsIndex_r4/Relational  mode=a!=b  en=off  latency=0  dbl_ovrd=off  block_type=relational
      settings: block_version=8.2
  Relational3 : xbsIndex_r4/Relational  mode=a=b  en=off  latency=0  dbl_ovrd=off  block_type=relational
      settings: block_version=8.2
  Relational4 : xbsIndex_r4/Relational  mode=a=b  en=off  latency=0  dbl_ovrd=off  block_type=relational
      settings: block_version=8.2
  WE : Outport
  RE : Outport  Port=2
  RST : Outport  Port=3
  Out_En : Outport  Port=4
  wires:
  Logical1/1 -> Out_En/1
  Logical2/1 -> RE/1
  Enable/1 -> Delay1/1, Logical2/1
  Counter/1 -> Relational3/1
  Relational3/1 -> Counter1/2, Logical3/1
  Counter1/1 -> Relational4/1, Relational/2, Relational1/1
  N/1 -> Relational4/2, AddSub/1
  Relational4/1 -> RST/1, Logical4/1
  Relational/1 -> Logical/1
  Logical/1 -> WE/1, Inverter/1
  Inverter/1 -> Logical1/1
  Constant/1 -> Relational1/2
  Relational1/1 -> Logical2/2
  Delay1/1 -> Counter/2, Logical/2, Logical1/2
  Constant1/1 -> AddSub/2
  Constant2/1 -> AddSub1/2
  AddSub1/1 -> Relational3/2
  M/1 -> AddSub1/1
  AddSub/1 -> Relational/1
  Logical3/1 -> Counter/1
  Reset/1 -> Logical3/2, Logical4/2
  Logical4/1 -> Counter1/1

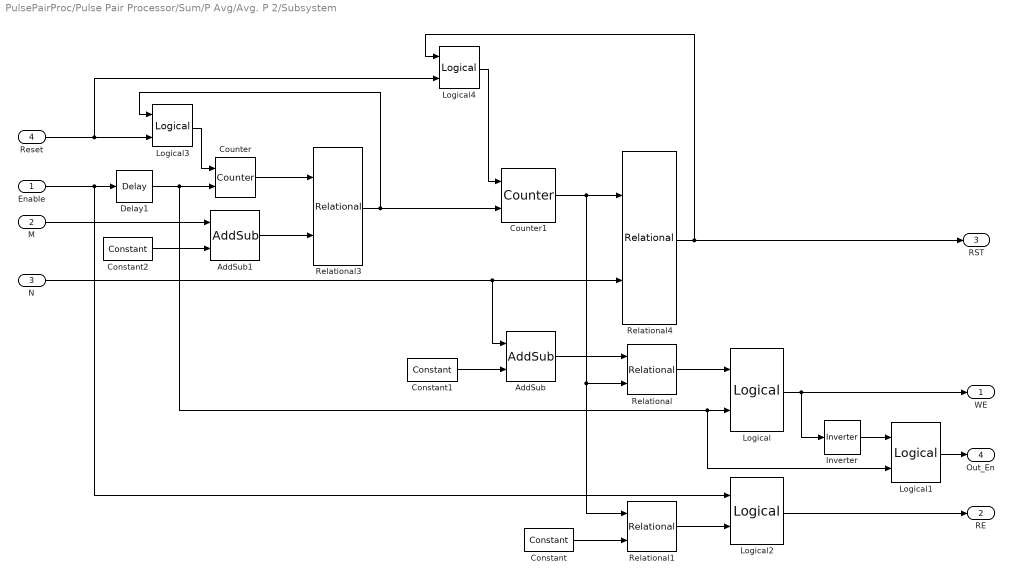
== system PulsePairProc/Pulse Pair Processor/Sum/P Avg/Avg. P 2/Subsystem ==
  Enable : Inport
  M : Inport  Port=2
  N : Inport  Port=3
  Reset : Inport  Port=4
  AddSub : xbsIndex_r4/AddSub  mode=Subtraction  use_carryin=off  use_carryout=off  en=off  latency=0  precision=User Defined  arith_type=Unsigned  n_bits=7  bin_pt=0  quantization="Round  (unbiased: +/- Inf)"  overflow=Flag as error  dbl_ovrd=off  use_behavioral_HDL=off  pipelined=off  use_rpm=on  block_type=addsub
      settings: block_version=8.2
  AddSub1 : xbsIndex_r4/AddSub  mode=Subtraction  use_carryin=off  use_carryout=off  en=off  latency=0  precision=User Defined  arith_type=Unsigned  n_bits=11  bin_pt=0  quantization="Round  (unbiased: +/- Inf)"  overflow=Flag as error  dbl_ovrd=off  use_behavioral_HDL=off  pipelined=off  use_rpm=on  block_type=addsub
      settings: block_version=8.2
  Constant : xbsIndex_r4/Constant  arith_type=Unsigned  const=0  n_bits=1  bin_pt=0  explicit_period=off  period=1  equ=P=C  opselect=C  inp2=PCIN>>17  opr=+  inp1=P  carry=CIN  dbl_ovrd=off  block_type=constant
      settings: block_version=8.2
  Constant1 : xbsIndex_r4/Constant  arith_type=Unsigned  const=1  n_bits=1  bin_pt=0  explicit_period=off  period=1  equ=P=C  opselect=C  inp2=PCIN>>17  opr=+  inp1=P  carry=CIN  dbl_ovrd=off  block_type=constant
      settings: block_version=8.2
  Constant2 : xbsIndex_r4/Constant  arith_type=Unsigned  const=1  n_bits=1  bin_pt=0  explicit_period=off  period=1  equ=P=C  opselect=C  inp2=PCIN>>17  opr=+  inp1=P  carry=CIN  dbl_ovrd=off  block_type=constant
      settings: block_version=8.2
  Counter : xbsIndex_r4/Counter  cnt_type=Free Running  cnt_to=11  operation=Up  start_count=0  cnt_by_val=1  arith_type=Unsigned  n_bits=11  bin_pt=0  load_pin=off  rst=on  en=on  explicit_period=on  period=1/12e6  dbl_ovrd=off  use_behavioral_HDL=off  use_rpm=off  block_type=counter
      settings: block_version=8.2
  Counter1 : xbsIndex_r4/Counter  cnt_type=Free Running  cnt_to=Inf  operation=Up  start_count=0  cnt_by_val=1  arith_type=Unsigned  n_bits=7  bin_pt=0  load_pin=off  rst=on  en=on  explicit_period=on  period=1/12e6  dbl_ovrd=off  use_behavioral_HDL=off  use_rpm=off  block_type=counter
      settings: block_version=8.2
  Delay1 : xbsIndex_r4/Delay  en=off  latency=1  dbl_ovrd=off  reg_retiming=off  block_type=delay
      settings: infoedit=Hardware notes: A delay line is a chain, each link of which is an SRL16 followed by a flip-flop. If register retiming is enabled, the delay line is a chain of flip-flops.  block_version=8.2
  Inverter : xbsIndex_r4/Inverter  en=off  latency=0  dbl_ovrd=off  block_type=inv
      settings: block_version=8.2
  Logical : xbsIndex_r4/Logical  logical_function=AND  inputs=2  en=off  latency=0  precision=Full  arith_type=Unsigned  n_bits=16  bin_pt=0  align_bp=on  dbl_ovrd=off  block_type=logical
      settings: block_version=8.2
  Logical1 : xbsIndex_r4/Logical  logical_function=AND  inputs=2  en=off  latency=0  precision=Full  arith_type=Unsigned  n_bits=16  bin_pt=0  align_bp=on  dbl_ovrd=off  block_type=logical
      settings: block_version=8.2
  Logical2 : xbsIndex_r4/Logical  logical_function=AND  inputs=2  en=off  latency=0  precision=Full  arith_type=Unsigned  n_bits=16  bin_pt=0  align_bp=on  dbl_ovrd=off  block_type=logical
      settings: block_version=8.2
  Logical3 : xbsIndex_r4/Logical  logical_function=OR  inputs=2  en=off  latency=0  precision=Full  arith_type=Unsigned  n_bits=16  bin_pt=0  align_bp=on  dbl_ovrd=off  block_type=logical
      settings: block_version=8.2
  Logical4 : xbsIndex_r4/Logical  logical_function=OR  inputs=2  en=off  latency=0  precision=Full  arith_type=Unsigned  n_bits=16  bin_pt=0  align_bp=on  dbl_ovrd=off  block_type=logical
      settings: block_version=8.2
  Relational : xbsIndex_r4/Relational  mode=a!=b  en=off  latency=0  dbl_ovrd=off  block_type=relational
      settings: block_version=8.2
  Relational1 : xbsIndex_r4/Relational  mode=a!=b  en=off  latency=0  dbl_ovrd=off  block_type=relational
      settings: block_version=8.2
  Relational3 : xbsIndex_r4/Relational  mode=a=b  en=off  latency=0  dbl_ovrd=off  block_type=relational
      settings: block_version=8.2
  Relational4 : xbsIndex_r4/Relational  mode=a=b  en=off  latency=0  dbl_ovrd=off  block_type=relational
      settings: block_version=8.2
  WE : Outport
  RE : Outport  Port=2
  RST : Outport  Port=3
  Out_En : Outport  Port=4
  wires:
  Logical1/1 -> Out_En/1
  Logical2/1 -> RE/1
  Enable/1 -> Delay1/1, Logical2/1
  Counter/1 -> Relational3/1
  Relational3/1 -> Counter1/2, Logical3/1
  Counter1/1 -> Relational4/1, Relational/2, Relational1/1
  N/1 -> Relational4/2, AddSub/1
  Relational4/1 -> RST/1, Logical4/1
  Relational/1 -> Logical/1
  Logical/1 -> WE/1, Inverter/1
  Inverter/1 -> Logical1/1
  Constant/1 -> Relational1/2
  Relational1/1 -> Logical2/2
  Delay1/1 -> Counter/2, Logical/2, Logical1/2
  Constant1/1 -> AddSub/2
  Constant2/1 -> AddSub1/2
  AddSub1/1 -> Relational3/2
  M/1 -> AddSub1/1
  AddSub/1 -> Relational/1
  Logical3/1 -> Counter/1
  Reset/1 -> Logical3/2, Logical4/2
  Logical4/1 -> Counter1/1
